simulink library "ADSB_Block"  (R2018b)
settings: Solver=VariableStepAuto  StartTime=0.0  StopTime=10.0  RelTol=1e-3
undefined symbols (not defined in the file): ac1dyn_alt0_ft, ac1dyn_lat0_rad, ac1dyn_lon0_rad, magnitude, uas_adsb_altQuant_ft, uas_adsb_avionicsSeed, uas_adsb_dt_s, uas_adsb_E_bias_ft, uas_adsb_E_random_stddev_ft, uas_adsb_E_tau_s, uas_adsb_Edot_bias_ftps, uas_adsb_Edot_random_stddev_ftps, uas_adsb_Edot_tau_s, uas_adsb_N_bias_ft, uas_adsb_N_random_stddev_ft, uas_adsb_N_tau_s, uas_adsb_Ndot_bias_ftps, uas_adsb_Ndot_random_stddev_ftps, uas_adsb_Ndot_tau_s, uas_adsb_probOneHit_3sec, uas_adsb_probOneHit_7sec, uas_adsb_randProbSeed, uas_adsb_rangeThreshold_ft, uas_adsb_reported_errorCovNED, uas_adsb_seed1, uas_adsb_seed2, uas_adsb_seed3, uas_adsb_seed4, uas_adsb_seed5, uas_adsb_seed6, uas_adsb_seed7, uas_adsb_sns_max_range_ft, uas_adsb_usePerfectAlt
libraries: simulink x7, TSAA_AltRate_Error x1, TSAA_Altitude_Error x1, CreateCovDiagMatrix x1, ExtractCovDiag x1
settings Model: Creator=RA24876  LastModifiedBy=BI28030
settings SFSimCC: SimUseLocalCustomCode=off
settings RTWCC: RTWUseLocalCustomCode=off
settings CodeAppCC: StateflowObjectComments=on

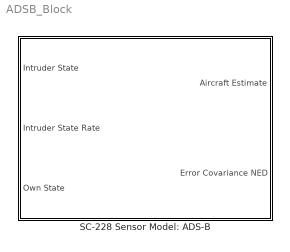
== system ADSB_Block ==
  SC-228 Sensor Model: ADS-B : Subsystem  mask(Tracked Surveillance: ADS-B){var_prefix=int_, dt_s=uas_adsb_dt_s, lat0_rad=ac1dyn_lat0_rad, lon0_rad=ac1dyn_lon0_rad, alt0_ft=ac1dyn_alt0_ft, avionicsSeed=uas_adsb_avionicsSeed, N_random_stddev_ft=uas_adsb_N_random_stddev_ft, N_bias_ft=uas_adsb_N_bias_ft, N_tau_s=uas_adsb_N_tau_s, seed1=uas_adsb_seed1, E_random_stddev_ft=uas_adsb_E_random_stddev_ft, E_bias_ft=uas_adsb_E_bias_ft, E_tau_s=uas_adsb_E_tau_s, seed2=uas_adsb_seed2, Ndot_random_stddev_ftps=uas_adsb_Ndot_random_stddev_ftps, Ndot_bias_ftps=uas_adsb_Ndot_bias_ftps, Ndot_tau_s=uas_adsb_Ndot_tau_s, seed5=uas_adsb_seed5, Edot_random_stddev_ftps=uas_adsb_Edot_random_stddev_ftps, Edot_bias_ftps=uas_adsb_Edot_bias_ftps, Edot_tau_s=uas_adsb_Edot_tau_s, seed6=uas_adsb_seed6, covNED=uas_adsb_reported_errorCovNED, perfect=uas_adsb_usePerfectAlt, seed3=uas_adsb_seed3, seed4=uas_adsb_seed4, altQuant_ft=uas_adsb_altQuant_ft, seed7=uas_adsb_seed7, sns_max_range_ft=uas_adsb_sns_max_range_ft, probOneHit_3sec=uas_adsb_probOneHit_3sec, probOneHit_7sec=uas_adsb_probOneHit_7sec, randProbSeed=uas_adsb_randProbSeed, rangeThreshold_ft=uas_adsb_rangeThreshold_ft}
      mask prompts: var_prefix "Variable Prefix"; dt_s "Timestep"; lat0_rad "ENU Origin Latitude"; lon0_rad "ENU Origin Longitude"; alt0_ft "ENU Origin Altitude"; avionicsSeed "Avionics Delay Seed"; N_random_stddev_ft "North Position Random Error Standard Deviation (ft)"; N_bias_ft "North Position Bias (ft)"; N_tau_s "Correlation Time (s)"; seed1 "Random Seed"; E_random_stddev_ft "East Position Random Error Standard Deviation (ft)"; E_bias_ft "East Position Bias (ft)"; E_tau_s "Correlation Time (s)"; seed2 "Random Seed"; Ndot_random_stddev_ftps "North Velocity Random Error Standard Deviation (ft/s)"; Ndot_bias_ftps "North Velocity Bias (ft/s)"; Ndot_tau_s "Correlation Time (s)"; seed5 "Random Seed"; Edot_random_stddev_ftps "East Velocity Random Error Standard Deviation (ft/s)"; Edot_bias_ftps "East Velocity Bias (ft/s)"; Edot_tau_s "Correlation Time (s)"; seed6 "Random Seed"; covNED "Error Covariance"; perfect "Use Perfect Altimetry"; seed3 "Lambda Random Seed"; seed4 "Random Seed"; altQuant_ft "Altitude Quantization (ft)"; seed7 "Lambda Random Seed"; sns_max_range_ft "Max Detection Range"; probOneHit_3sec "Single Hit Probability (95% detection in 3 sec)"; probOneHit_7sec "Single Hit Probability (95% detection in 7 sec)"; randProbSeed "Random Seed"; rangeThreshold_ft "Range at which detection probabilities change"
      mask help: Additive noise model of ADS-B
      mask init:
      | set_param( [ gcb '/To Workspace' ], 'VariableName', [ var_prefix 'uncompDelay' ] )
      mask Help:
      | Additive noise model of ADS-B. Independent noise is added to each
      | position and velocity component in a North-East-Down coordinate system.
      | Noise is colored using weights determined by time constant parameters.
      | 
      | Output takes the form of a AircraftEstimate data bus and a 6x6 error covariance
      | matrix in North-East-Down.
      mask DialogControl ParameterTabVar0 Prompt: General
      mask DialogControl ParameterTabVar01 Prompt: Position (N)
      mask DialogControl ParameterTabVar012 Prompt: Position (E)
      mask DialogControl ParameterTabVar01234 Prompt: Velocity (N)
      mask DialogControl ParameterTabVar012345 Prompt: Velocity (E)
      mask DialogControl ParameterTabVar01234567 Prompt: Covariance
      mask DialogControl ParameterTabVar012345678 Prompt: Altitude
      mask DialogControl ParameterTabVar0123456789 Prompt: Vertical Rate
      mask DialogControl ParameterTabVar012345678910 Prompt: Detection

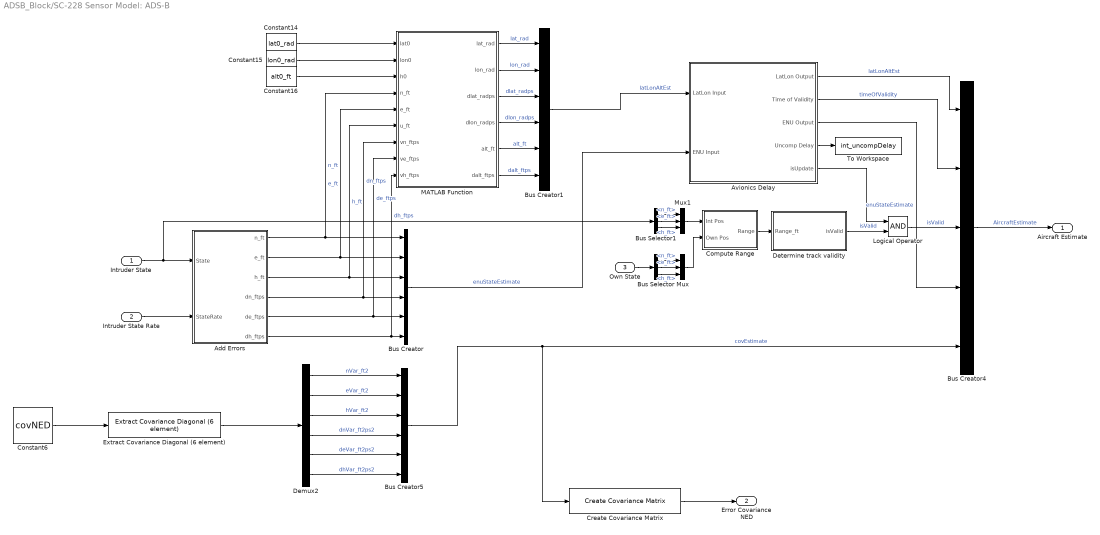
== system ADSB_Block/SC-228 Sensor Model: ADS-B ==
  Intruder State : Inport  OutDataTypeStr=Bus: AircraftState
  Intruder State Rate : Inport  Port=2  OutDataTypeStr=Bus: AircraftStateRate
  Own State : Inport  Port=3  OutDataTypeStr=Bus: AircraftState
  Add Errors : Subsystem
  Avionics Delay : Subsystem  mask{dt=dt_s, seed2=avionicsSeed}
      mask prompts: dt "Sample Time (s)"; seed2 "RNG Seed"
  Bus Creator : BusCreator  Inputs=6  OutDataTypeStr=Bus: StateEstimate
  Bus Creator1 : BusCreator  Inputs=6  OutDataTypeStr=Bus: LatLonAltMeasurement
  Bus Creator4 : BusCreator  Inputs='latLonAltEst','timeOfValidity','isValid','enuStateEstimate','covEstimate'  OutDataTypeStr=Bus: AircraftEstimate  NonVirtualBus=on
  Bus Creator5 : BusCreator  Inputs=6  OutDataTypeStr=Bus: CovarianceEstimate
  Bus Selector : BusSelector  OutputSignals=n_ft,e_ft,h_ft
  Bus Selector1 : BusSelector  OutputSignals=n_ft,e_ft,h_ft
  Compute Range : Subsystem
  Constant14 : Constant  Value=lat0_rad  OutDataTypeStr=double
  Constant15 : Constant  Value=lon0_rad  OutDataTypeStr=double
  Constant16 : Constant  Value=alt0_ft  OutDataTypeStr=double
  Constant6 : Constant  Value=covNED
  Create Covariance Matrix : CreateCovDiagMatrix/Create Covariance Matrix  SystemSampleTime=-1
  Demux2 : Demux  Outputs=6
  Determine track validity : Subsystem  mask{sns_max_range_ft=sns_max_range_ft, probOneHit_3sec=probOneHit_3sec, probOneHit_7sec=probOneHit_7sec, randProbSeed=randProbSeed, rangeThreshold_ft=rangeThreshold_ft}
      mask prompts: sns_max_range_ft "Max Detection Range (ft)"; probOneHit_3sec "Probability of a Single Hit (95% Detection in 3 sec)"; probOneHit_7sec "Probability of a Single Hit (95% Detection in 7 sec)"; randProbSeed "Random Seed"; rangeThreshold_ft "Range Where Detection Probabilites Change"
  Extract Covariance Diagonal (6 element) : ExtractCovDiag/Extract Covariance Diagonal (6 element)  SystemSampleTime=-1
  Logical Operator : Logic  AllPortsSameDT=off  OutDataTypeStr=boolean
  MATLAB Function : MATLAB Function  TreatAsAtomicUnit=on
  Mux : Mux  Inputs=3
  Mux1 : Mux  Inputs=3
  To Workspace : ToWorkspace  VariableName=int_uncompDelay  SaveFormat=Timeseries  SampleTime=-1
  Aircraft Estimate : Outport  OutDataTypeStr=Bus: AircraftEstimate
  Error Covariance NED : Outport  Port=2
  wires:
  Avionics Delay/5(isUpdate) -> Logical Operator/1
  Logical Operator/1 -> Bus Creator4/3  "isValid"
  Mux1/1 -> Compute Range/1(Int Pos)
  Bus Selector1/3 -> Mux1/3  "<h_ft>"
  Bus Selector1/2 -> Mux1/2  "<e_ft>"
  Bus Selector1/1 -> Mux1/1  "<n_ft>"
  Intruder State/1 -> Add Errors/1(State), Bus Selector1/1
  Mux/1 -> Compute Range/2(Own Pos)
  Bus Selector/3 -> Mux/3  "<h_ft>"
  Bus Selector/2 -> Mux/2  "<e_ft>"
  Bus Selector/1 -> Mux/1  "<n_ft>"
  Own State/1 -> Bus Selector/1
  Bus Creator4/1 -> Aircraft Estimate/1  "AircraftEstimate"
  Bus Creator5/1 -> Create Covariance Matrix/1, Bus Creator4/5  "covEstimate"
  MATLAB Function/6(dalt_ftps) -> Bus Creator1/6  "dalt_ftps"
  MATLAB Function/5(alt_ft) -> Bus Creator1/5  "alt_ft"
  MATLAB Function/4(dlon_radps) -> Bus Creator1/4  "dlon_radps"
  MATLAB Function/3(dlat_radps) -> Bus Creator1/3  "dlat_radps"
  MATLAB Function/2(lon_rad) -> Bus Creator1/2  "lon_rad"
  MATLAB Function/1(lat_rad) -> Bus Creator1/1  "lat_rad"
  Bus Creator1/1 -> Avionics Delay/1(LatLon Input)  "latLonAltEst"
  Constant14/1 -> MATLAB Function/1(lat0)
  Constant16/1 -> MATLAB Function/3(h0)
  Constant15/1 -> MATLAB Function/2(lon0)
  Bus Creator/1 -> Avionics Delay/2(ENU Input)  "enuStateEstimate"
  Add Errors/1(n_ft) -> MATLAB Function/4(n_ft), Bus Creator/1  "n_ft"
  Add Errors/2(e_ft) -> MATLAB Function/5(e_ft), Bus Creator/2  "e_ft"
  Add Errors/3(h_ft) -> MATLAB Function/6(u_ft), Bus Creator/3  "h_ft"
  Add Errors/6(dh_ftps) -> MATLAB Function/9(vh_ftps), Bus Creator/6  "dh_ftps"
  Add Errors/4(dn_ftps) -> MATLAB Function/7(vn_ftps), Bus Creator/4  "dn_ftps"
  Add Errors/5(de_ftps) -> MATLAB Function/8(ve_ftps), Bus Creator/5  "de_ftps"
  Intruder State Rate/1 -> Add Errors/2(StateRate)
  Extract Covariance Diagonal (6 element)/1 -> Demux2/1
  Demux2/4 -> Bus Creator5/4  "dnVar_ft2ps2"
  Demux2/5 -> Bus Creator5/5  "deVar_ft2ps2"
  Demux2/2 -> Bus Creator5/2  "eVar_ft2"
  Demux2/1 -> Bus Creator5/1  "nVar_ft2"
  Constant6/1 -> Extract Covariance Diagonal (6 element)/1
  Compute Range/1(Range) -> Determine track validity/1(Range_ft)
  Determine track validity/1(isValid) -> Logical Operator/2  "isValid"
  Avionics Delay/3(ENU Output) -> Bus Creator4/4  "enuStateEstimate"
  Avionics Delay/2(Time of Validity) -> Bus Creator4/2  "timeOfValidity"
  Avionics Delay/4(Uncomp Delay) -> To Workspace/1
  Avionics Delay/1(LatLon Output) -> Bus Creator4/1  "latLonAltEst"
  Demux2/3 -> Bus Creator5/3  "hVar_ft2"
  Demux2/6 -> Bus Creator5/6  "dhVar_ft2ps2"
  Create Covariance Matrix/1 -> Error Covariance NED/1

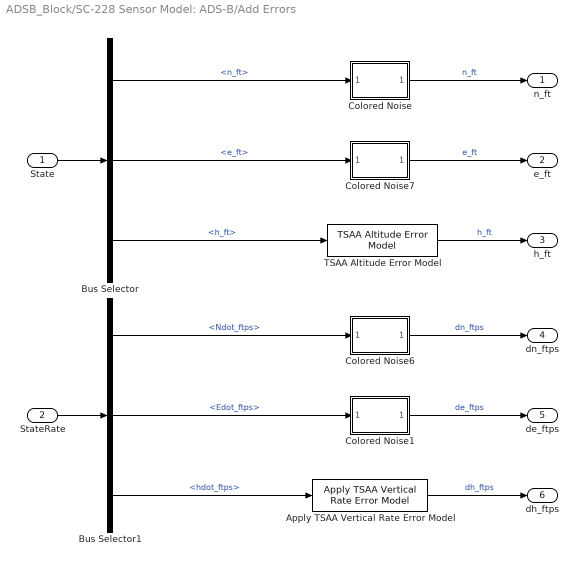
== system ADSB_Block/SC-228 Sensor Model: ADS-B/Add Errors ==
  State : Inport  OutDataTypeStr=Bus: AircraftState
  StateRate : Inport  Port=2  OutDataTypeStr=Bus: AircraftStateRate
  Apply TSAA Vertical Rate Error Model : TSAA_AltRate_Error/Apply TSAA Vertical Rate Error Model  perfect=perfect  seed=seed6  dt_s=dt_s
  Bus Selector : BusSelector  OutputSignals=n_ft,e_ft,h_ft
  Bus Selector1 : BusSelector  OutputSignals=Ndot_ftps,Edot_ftps,hdot_ftps
  Colored Noise : Subsystem  mask(Colored Noise){sig=N_random_stddev_ft, bias=N_bias_ft, tau=N_tau_s, dt=dt_s, seed=seed1}
      mask prompts: sig "Random error standard deviation"; bias "Bias error"; tau "Correlation time"; dt "Track update time"; seed "Random Seed"
      mask help: Generates a noisy state variable estimate using the ABSAA colored noise model. Set correlation time to zero for white noise.
      mask Help:
      | Generates a noisy state variable estimate using the AF Common ABSAA error
      | model.  Time correlation of the error is defined by an exponential decay
      | of K = exp(-tau/dt), where tau is the correlation time and dt is the time
      | between track updates.  The track error at time t is then:
      | 
      |     err(t) = K*err(t-1) + N(0,(1-K^2)*sig^2) + bias
      | 
      | where N(x,y) is a Gaussian noise process with mean x and variance y and
      | with random number generator seeded with the integer 'seed'.
      | 
      | The random noise process must be initialized with an error drawn from
      | N(0,sig^2).
      | 
      | The noise model can be used to produce white noise by setting tau to zero.
  Colored Noise1 : Subsystem  mask(Colored Noise){sig=Edot_random_stddev_ftps, bias=Edot_bias_ftps, tau=Edot_tau_s, dt=dt_s, seed=seed6}
      mask prompts: sig "Random error standard deviation"; bias "Bias error"; tau "Correlation time"; dt "Track update time"; seed "Random Seed"
      mask help: Generates a noisy state variable estimate using the ABSAA colored noise model. Set correlation time to zero for white noise.
      mask Help:
      | Generates a noisy state variable estimate using the AF Common ABSAA error
      | model.  Time correlation of the error is defined by an exponential decay
      | of K = exp(-tau/dt), where tau is the correlation time and dt is the time
      | between track updates.  The track error at time t is then:
      | 
      |     err(t) = K*err(t-1) + N(0,(1-K^2)*sig^2) + bias
      | 
      | where N(x,y) is a Gaussian noise process with mean x and variance y and
      | with random number generator seeded with the integer 'seed'.
      | 
      | The random noise process must be initialized with an error drawn from
      | N(0,sig^2).
      | 
      | The noise model can be used to produce white noise by setting tau to zero.
  Colored Noise6 : Subsystem  mask(Colored Noise){sig=Ndot_random_stddev_ftps, bias=Ndot_bias_ftps, tau=Ndot_tau_s, dt=dt_s, seed=seed5}
      mask prompts: sig "Random error standard deviation"; bias "Bias error"; tau "Correlation time"; dt "Track update time"; seed "Random Seed"
      mask help: Generates a noisy state variable estimate using the ABSAA colored noise model. Set correlation time to zero for white noise.
      mask Help:
      | Generates a noisy state variable estimate using the AF Common ABSAA error
      | model.  Time correlation of the error is defined by an exponential decay
      | of K = exp(-tau/dt), where tau is the correlation time and dt is the time
      | between track updates.  The track error at time t is then:
      | 
      |     err(t) = K*err(t-1) + N(0,(1-K^2)*sig^2) + bias
      | 
      | where N(x,y) is a Gaussian noise process with mean x and variance y and
      | with random number generator seeded with the integer 'seed'.
      | 
      | The random noise process must be initialized with an error drawn from
      | N(0,sig^2).
      | 
      | The noise model can be used to produce white noise by setting tau to zero.
  Colored Noise7 : Subsystem  mask(Colored Noise){sig=E_random_stddev_ft, bias=E_bias_ft, tau=E_tau_s, dt=dt_s, seed=seed2}
      mask prompts: sig "Random error standard deviation"; bias "Bias error"; tau "Correlation time"; dt "Track update time"; seed "Random Seed"
      mask help: Generates a noisy state variable estimate using the ABSAA colored noise model. Set correlation time to zero for white noise.
      mask Help:
      | Generates a noisy state variable estimate using the AF Common ABSAA error
      | model.  Time correlation of the error is defined by an exponential decay
      | of K = exp(-tau/dt), where tau is the correlation time and dt is the time
      | between track updates.  The track error at time t is then:
      | 
      |     err(t) = K*err(t-1) + N(0,(1-K^2)*sig^2) + bias
      | 
      | where N(x,y) is a Gaussian noise process with mean x and variance y and
      | with random number generator seeded with the integer 'seed'.
      | 
      | The random noise process must be initialized with an error drawn from
      | N(0,sig^2).
      | 
      | The noise model can be used to produce white noise by setting tau to zero.
  TSAA Altitude Error Model : TSAA_Altitude_Error/TSAA Altitude Error Model  ac_id=2  perfect=perfect  lambdaSeed=seed3  randomSeed=seed4  altQuant_ft=altQuant_ft  dt_s=dt_s
  n_ft : Outport
  e_ft : Outport  Port=2
  h_ft : Outport  Port=3
  dn_ftps : Outport  Port=4
  de_ftps : Outport  Port=5
  dh_ftps : Outport  Port=6
  wires:
  Bus Selector/3 -> TSAA Altitude Error Model/1  "<h_ft>"
  Bus Selector/1 -> Colored Noise/1(truth)  "<n_ft>"
  State/1 -> Bus Selector/1
  Colored Noise1/1(noisy) -> de_ftps/1  "de_ftps"
  Apply TSAA Vertical Rate Error Model/1 -> dh_ftps/1  "dh_ftps"
  Colored Noise6/1(noisy) -> dn_ftps/1  "dn_ftps"
  Colored Noise7/1(noisy) -> e_ft/1  "e_ft"
  Colored Noise/1(noisy) -> n_ft/1  "n_ft"
  Bus Selector/2 -> Colored Noise7/1(truth)  "<e_ft>"
  TSAA Altitude Error Model/1 -> h_ft/1  "h_ft"
  StateRate/1 -> Bus Selector1/1
  Bus Selector1/1 -> Colored Noise6/1(truth)  "<Ndot_ftps>"
  Bus Selector1/2 -> Colored Noise1/1(truth)  "<Edot_ftps>"
  Bus Selector1/3 -> Apply TSAA Vertical Rate Error Model/1  "<hdot_ftps>"

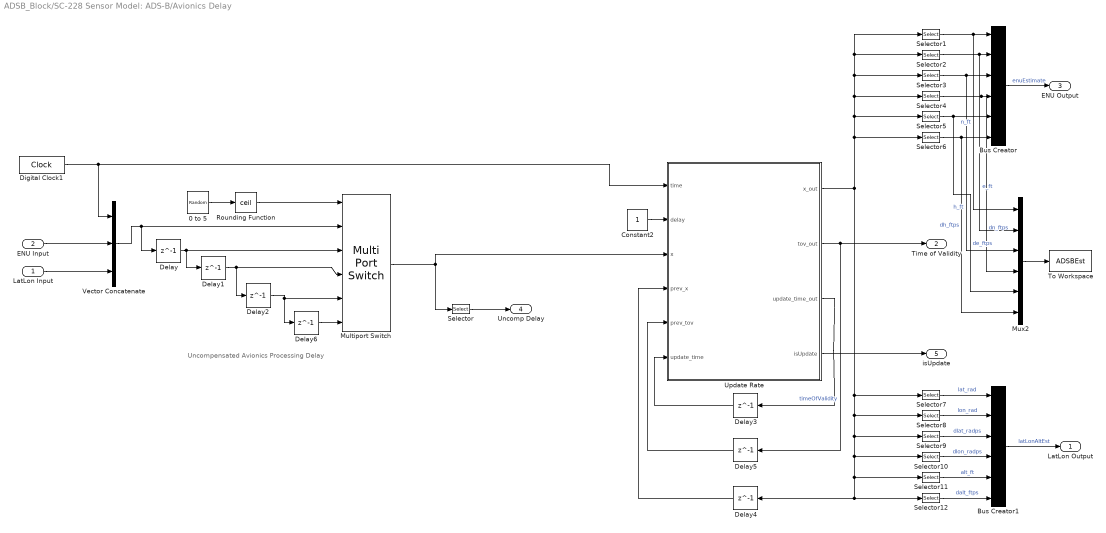
== system ADSB_Block/SC-228 Sensor Model: ADS-B/Avionics Delay ==
  note: Uncompensated Avionics Processing Delay
  LatLon Input : Inport
  ENU Input : Inport  Port=2
  0 to 5 : UniformRandomNumber  Minimum=0  Maximum=5  Seed=seed2  SampleTime=dt_s
  Bus Creator : BusCreator  Inputs=6
  Bus Creator1 : BusCreator  Inputs=6
  Constant2 : Constant
  Delay{,1..2,6} (4 alike) : Delay  DelayLength=1
  Delay3 : Delay  DelayLength=1  InitialCondition=1
  Delay4 : Delay  DelayLength=1  InitialCondition=0
  Delay5 : Delay  DelayLength=1  InitialCondition=0
  Digital Clock1 : DigitalClock  SampleTime=dt_s
  Multiport Switch : MultiPortSwitch  Inputs=5
  Mux2 : Mux  Inputs=6
  Rounding Function : Rounding  Operator=ceil
  Selector : Selector  InputPortWidth=13  IndexOptions=Index vector (dialog)  Indices=[1]  OutputSizes=1
  Selector1 : Selector  InputPortWidth=13  IndexOptions=Index vector (dialog)  Indices=[2]  OutputSizes=1
  Selector10 : Selector  InputPortWidth=13  IndexOptions=Index vector (dialog)  Indices=[11]  OutputSizes=1
  Selector11 : Selector  InputPortWidth=13  IndexOptions=Index vector (dialog)  Indices=[12]  OutputSizes=1
  Selector12 : Selector  InputPortWidth=13  IndexOptions=Index vector (dialog)  Indices=[13]  OutputSizes=1
  Selector2 : Selector  InputPortWidth=13  IndexOptions=Index vector (dialog)  Indices=[3]  OutputSizes=1
  Selector3 : Selector  InputPortWidth=13  IndexOptions=Index vector (dialog)  Indices=[4]  OutputSizes=1
  Selector4 : Selector  InputPortWidth=13  IndexOptions=Index vector (dialog)  Indices=[5]  OutputSizes=1
  Selector5 : Selector  InputPortWidth=13  IndexOptions=Index vector (dialog)  Indices=[6]  OutputSizes=1
  Selector6 : Selector  InputPortWidth=13  IndexOptions=Index vector (dialog)  Indices=[7]  OutputSizes=1
  Selector7 : Selector  InputPortWidth=13  IndexOptions=Index vector (dialog)  Indices=[8]  OutputSizes=1
  Selector8 : Selector  InputPortWidth=13  IndexOptions=Index vector (dialog)  Indices=[9]  OutputSizes=1
  Selector9 : Selector  InputPortWidth=13  IndexOptions=Index vector (dialog)  Indices=[10]  OutputSizes=1
  To Workspace : ToWorkspace  VariableName=ADSBEst  SampleTime=-1
  Update Rate : MATLAB Function  TreatAsAtomicUnit=on
  Vector Concatenate : Concatenate  NumInputs=3
  LatLon Output : Outport
  Time of Validity : Outport  Port=2
  ENU Output : Outport  Port=3
  Uncomp Delay : Outport  Port=4
  isUpdate : Outport  Port=5
  wires:
  Update Rate/4(isUpdate) -> isUpdate/1
  Constant2/1 -> Update Rate/2(delay)
  Selector1/1 -> Mux2/1, Bus Creator/1  "n_ft"
  Vector Concatenate/1 -> Delay/1, Multiport Switch/2
  Selector/1 -> Uncomp Delay/1
  ENU Input/1 -> Vector Concatenate/2
  Multiport Switch/1 -> Update Rate/3(x), Selector/1
  Delay5/1 -> Update Rate/5(prev_tov)
  Update Rate/2(tov_out) -> Time of Validity/1, Delay5/1  "timeOfValidity"
  Delay3/1 -> Update Rate/6(update_time)
  Delay4/1 -> Update Rate/4(prev_x)
  Update Rate/3(update_time_out) -> Delay3/1
  Digital Clock1/1 -> Update Rate/1(time), Vector Concatenate/1
  Rounding Function/1 -> Multiport Switch/1
  0 to 5/1 -> Rounding Function/1
  Delay/1 -> Multiport Switch/3, Delay1/1
  Delay1/1 -> Multiport Switch/4, Delay2/1
  Delay2/1 -> Multiport Switch/5, Delay6/1
  Selector2/1 -> Mux2/2, Bus Creator/2  "e_ft"
  Selector3/1 -> Mux2/3, Bus Creator/3  "h_ft"
  Selector4/1 -> Mux2/4, Bus Creator/4  "dn_ftps"
  Selector5/1 -> Mux2/5, Bus Creator/5  "de_ftps"
  Selector6/1 -> Mux2/6, Bus Creator/6  "dh_ftps"
  Bus Creator/1 -> ENU Output/1  "enuEstimate"
  Delay6/1 -> Multiport Switch/6
  LatLon Input/1 -> Vector Concatenate/3
  Bus Creator1/1 -> LatLon Output/1  "latLonAltEst"
  Update Rate/1(x_out) -> Selector7/1, Delay4/1, Selector12/1, Selector11/1, Selector10/1, Selector9/1, Selector8/1, Selector6/1, Selector5/1, Selector4/1, Selector3/1, Selector2/1, Selector1/1
  Selector12/1 -> Bus Creator1/6  "dalt_ftps"
  Selector7/1 -> Bus Creator1/1  "lat_rad"
  Selector8/1 -> Bus Creator1/2  "lon_rad"
  Selector11/1 -> Bus Creator1/5  "alt_ft"
  Selector10/1 -> Bus Creator1/4  "dlon_radps"
  Selector9/1 -> Bus Creator1/3  "dlat_radps"
  Mux2/1 -> To Workspace/1

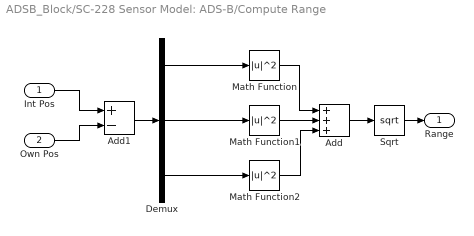
== system ADSB_Block/SC-228 Sensor Model: ADS-B/Compute Range ==
  Int Pos : Inport
  Own Pos : Inport  Port=2
  Add : Sum  Inputs=+++
  Add1 : Sum  Inputs=+-
  Demux : Demux  Outputs=3
  Math Function : Math  Operator=magnitude^2  SaturateOnIntegerOverflow=on
  Math Function1 : Math  Operator=magnitude^2  SaturateOnIntegerOverflow=on
  Math Function2 : Math  Operator=magnitude^2  SaturateOnIntegerOverflow=on
  Sqrt : Sqrt  SaturateOnIntegerOverflow=on
  Range : Outport
  wires:
  Demux/3 -> Math Function2/1
  Demux/1 -> Math Function/1
  Demux/2 -> Math Function1/1
  Add1/1 -> Demux/1
  Own Pos/1 -> Add1/2
  Int Pos/1 -> Add1/1
  Math Function/1 -> Add/1
  Sqrt/1 -> Range/1
  Math Function1/1 -> Add/2
  Add/1 -> Sqrt/1
  Math Function2/1 -> Add/3

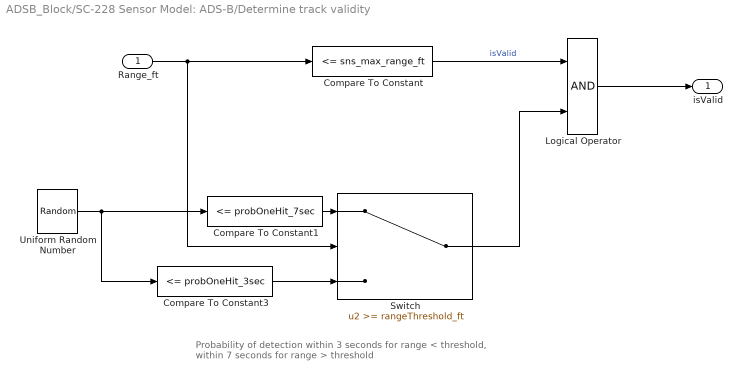
== system ADSB_Block/SC-228 Sensor Model: ADS-B/Determine track validity ==
  note: Probability of detection within 3 seconds for range < threshold,
      | within 7 seconds for range > threshold
  Range_ft : Inport
  Compare To Constant : simulink/Logic and Bit Operations/Compare To Constant  relop=<=  const=sns_max_range_ft  OutDataTypeStr=boolean
  Compare To Constant1 : simulink/Logic and Bit Operations/Compare To Constant  relop=<=  const=probOneHit_7sec  OutDataTypeStr=boolean
  Compare To Constant3 : simulink/Logic and Bit Operations/Compare To Constant  relop=<=  const=probOneHit_3sec  OutDataTypeStr=boolean
  Logical Operator : Logic  AllPortsSameDT=off  OutDataTypeStr=boolean
  Switch : Switch  Threshold=rangeThreshold_ft
  Uniform Random Number : UniformRandomNumber  Minimum=0  Seed=randProbSeed  SampleTime=dt_s
  isValid : Outport
  wires:
  Range_ft/1 -> Compare To Constant/1, Switch/2
  Compare To Constant/1 -> Logical Operator/1  "isValid"
  Logical Operator/1 -> isValid/1
  Switch/1 -> Logical Operator/2
  Compare To Constant1/1 -> Switch/1
  Uniform Random Number/1 -> Compare To Constant3/1, Compare To Constant1/1
  Compare To Constant3/1 -> Switch/3

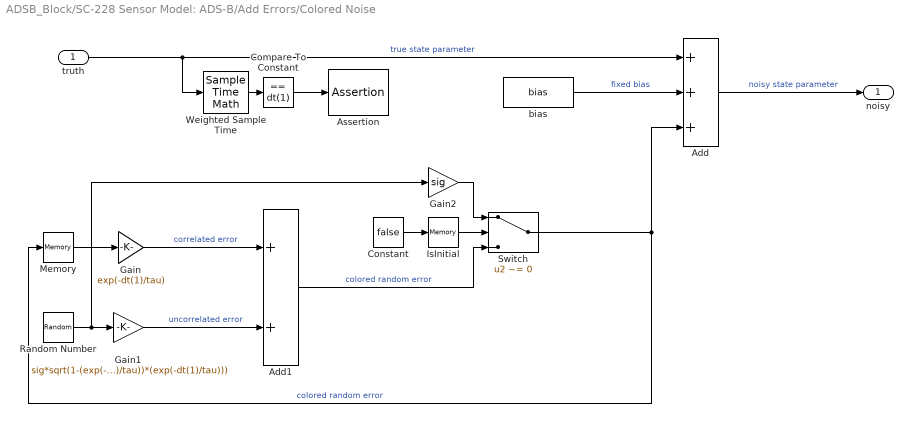
== system ADSB_Block/SC-228 Sensor Model: ADS-B/Add Errors/Colored Noise ==
  truth : Inport
  Add : Sum  Inputs=+++
  Add1 : Sum
  Assertion : Assertion
  Compare To Constant : simulink/Logic and Bit Operations/Compare To Constant  relop===  const=dt(1)  OutDataTypeStr=boolean
  Constant : Constant  Value=false
  Gain : Gain  Gain=exp(-dt(1)/tau)
  Gain1 : Gain  Gain=sig*sqrt(1-(exp(-dt(1)/tau))*(exp(-dt(1)/tau)))
  Gain2 : Gain  Gain=sig
  IsInitial : Memory  InitialCondition=true  InheritSampleTime=on
  Memory : Memory  InheritSampleTime=on
  Random Number : RandomNumber  Seed=seed  SampleTime=dt_s
  Switch : Switch  Criteria=u2 ~= 0
  Weighted Sample Time : SampleTimeMath  TsampMathOp=Ts Only
  bias : Constant  Value=bias
  noisy : Outport
  wires:
  Compare To Constant/1 -> Assertion/1
  Weighted Sample Time/1 -> Compare To Constant/1
  Gain2/1 -> Switch/1
  Add1/1 -> Switch/3  "colored random error"
  IsInitial/1 -> Switch/2
  Constant/1 -> IsInitial/1
  Memory/1 -> Gain/1
  truth/1 -> Add/1, Weighted Sample Time/1  "true state parameter"
  Add/1 -> noisy/1  "noisy state parameter"
  Gain/1 -> Add1/1  "correlated error"
  Random Number/1 -> Gain1/1, Gain2/1
  bias/1 -> Add/2  "fixed bias"
  Switch/1 -> Add/3, Memory/1  "colored random error"
  Gain1/1 -> Add1/2  "uncorrelated error"

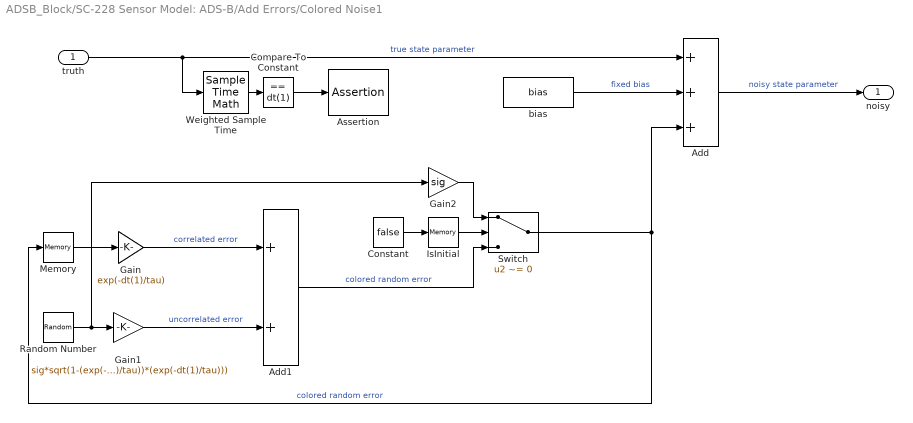
== system ADSB_Block/SC-228 Sensor Model: ADS-B/Add Errors/Colored Noise1 ==
  truth : Inport
  Add : Sum  Inputs=+++
  Add1 : Sum
  Assertion : Assertion
  Compare To Constant : simulink/Logic and Bit Operations/Compare To Constant  relop===  const=dt(1)  OutDataTypeStr=boolean
  Constant : Constant  Value=false
  Gain : Gain  Gain=exp(-dt(1)/tau)
  Gain1 : Gain  Gain=sig*sqrt(1-(exp(-dt(1)/tau))*(exp(-dt(1)/tau)))
  Gain2 : Gain  Gain=sig
  IsInitial : Memory  InitialCondition=true  InheritSampleTime=on
  Memory : Memory  InheritSampleTime=on
  Random Number : RandomNumber  Seed=seed  SampleTime=dt_s
  Switch : Switch  Criteria=u2 ~= 0
  Weighted Sample Time : SampleTimeMath  TsampMathOp=Ts Only
  bias : Constant  Value=bias
  noisy : Outport
  wires:
  Compare To Constant/1 -> Assertion/1
  Weighted Sample Time/1 -> Compare To Constant/1
  Gain2/1 -> Switch/1
  Add1/1 -> Switch/3  "colored random error"
  IsInitial/1 -> Switch/2
  Constant/1 -> IsInitial/1
  Memory/1 -> Gain/1
  truth/1 -> Add/1, Weighted Sample Time/1  "true state parameter"
  Add/1 -> noisy/1  "noisy state parameter"
  Gain/1 -> Add1/1  "correlated error"
  Random Number/1 -> Gain1/1, Gain2/1
  bias/1 -> Add/2  "fixed bias"
  Switch/1 -> Add/3, Memory/1  "colored random error"
  Gain1/1 -> Add1/2  "uncorrelated error"

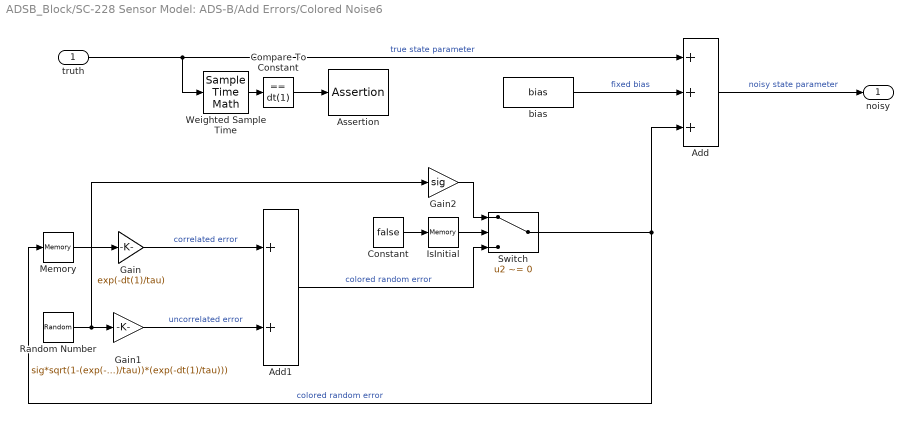
== system ADSB_Block/SC-228 Sensor Model: ADS-B/Add Errors/Colored Noise6 ==
  truth : Inport
  Add : Sum  Inputs=+++
  Add1 : Sum
  Assertion : Assertion
  Compare To Constant : simulink/Logic and Bit Operations/Compare To Constant  relop===  const=dt(1)  OutDataTypeStr=boolean
  Constant : Constant  Value=false
  Gain : Gain  Gain=exp(-dt(1)/tau)
  Gain1 : Gain  Gain=sig*sqrt(1-(exp(-dt(1)/tau))*(exp(-dt(1)/tau)))
  Gain2 : Gain  Gain=sig
  IsInitial : Memory  InitialCondition=true  InheritSampleTime=on
  Memory : Memory  InheritSampleTime=on
  Random Number : RandomNumber  Seed=seed  SampleTime=dt_s
  Switch : Switch  Criteria=u2 ~= 0
  Weighted Sample Time : SampleTimeMath  TsampMathOp=Ts Only
  bias : Constant  Value=bias
  noisy : Outport
  wires:
  Compare To Constant/1 -> Assertion/1
  Weighted Sample Time/1 -> Compare To Constant/1
  Gain2/1 -> Switch/1
  Add1/1 -> Switch/3  "colored random error"
  IsInitial/1 -> Switch/2
  Constant/1 -> IsInitial/1
  Memory/1 -> Gain/1
  truth/1 -> Add/1, Weighted Sample Time/1  "true state parameter"
  Add/1 -> noisy/1  "noisy state parameter"
  Gain/1 -> Add1/1  "correlated error"
  Random Number/1 -> Gain1/1, Gain2/1
  bias/1 -> Add/2  "fixed bias"
  Switch/1 -> Add/3, Memory/1  "colored random error"
  Gain1/1 -> Add1/2  "uncorrelated error"

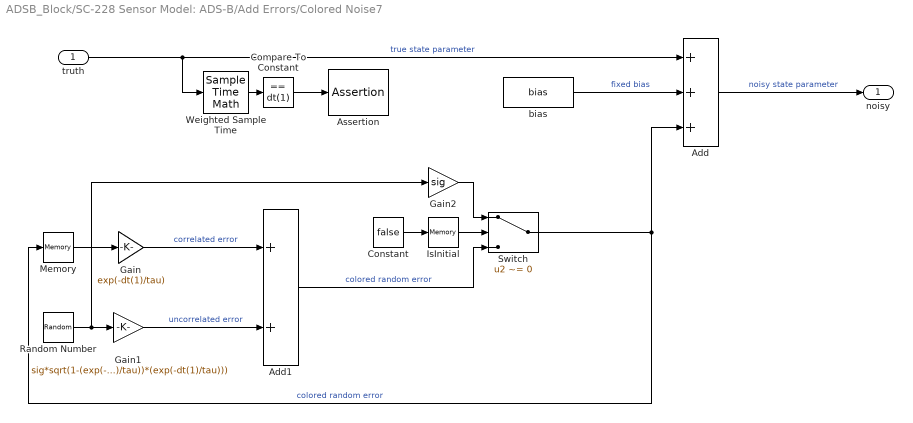
== system ADSB_Block/SC-228 Sensor Model: ADS-B/Add Errors/Colored Noise7 ==
  truth : Inport
  Add : Sum  Inputs=+++
  Add1 : Sum
  Assertion : Assertion
  Compare To Constant : simulink/Logic and Bit Operations/Compare To Constant  relop===  const=dt(1)  OutDataTypeStr=boolean
  Constant : Constant  Value=false
  Gain : Gain  Gain=exp(-dt(1)/tau)
  Gain1 : Gain  Gain=sig*sqrt(1-(exp(-dt(1)/tau))*(exp(-dt(1)/tau)))
  Gain2 : Gain  Gain=sig
  IsInitial : Memory  InitialCondition=true  InheritSampleTime=on
  Memory : Memory  InheritSampleTime=on
  Random Number : RandomNumber  Seed=seed  SampleTime=dt_s
  Switch : Switch  Criteria=u2 ~= 0
  Weighted Sample Time : SampleTimeMath  TsampMathOp=Ts Only
  bias : Constant  Value=bias
  noisy : Outport
  wires:
  Gain1/1 -> Add1/2  "uncorrelated error"
  Switch/1 -> Memory/1, Add/3  "colored random error"
  bias/1 -> Add/2  "fixed bias"
  Random Number/1 -> Gain2/1, Gain1/1
  Gain/1 -> Add1/1  "correlated error"
  Add/1 -> noisy/1  "noisy state parameter"
  truth/1 -> Weighted Sample Time/1, Add/1  "true state parameter"
  Memory/1 -> Gain/1
  Constant/1 -> IsInitial/1
  IsInitial/1 -> Switch/2
  Add1/1 -> Switch/3  "colored random error"
  Gain2/1 -> Switch/1
  Weighted Sample Time/1 -> Compare To Constant/1
  Compare To Constant/1 -> Assertion/1

== matlab function ADSB_Block/SC-228 Sensor Model: ADS-B/Avionics Delay/Update Rate ==
  data: time input; x_out output; tov_out output; delay input; x input; prev_x input; prev_tov input; update_time input; update_time_out output; isUpdate output
function [x_out,tov_out,update_time_out,isUpdate] = fcn(time,delay,x,prev_x,prev_tov,update_time)
%#codegen

if time-update_time>=-0.001 % pass out new output
    update_time_out = time+delay; 
    x_out = x;
    tov_out = time;
    isUpdate = true;
else % continue passing out old output
    x_out = prev_x; 
    update_time_out = update_time;
    tov_out = prev_tov;
    isUpdate = false;
end

== matlab function ADSB_Block/SC-228 Sensor Model: ADS-B/MATLAB Function ==
  data: lat0 input double; lon0 input double; h0 input double; n_ft input double; e_ft input double size=1; u_ft input double; vn_ftps input double; ve_ftps input double; vh_ftps input double; lat_rad output double; lon_rad output double; dlat_radps output double; dlon_radps output double; alt_ft output double; dalt_ftps output double
function [lat_rad,lon_rad,dlat_radps,dlon_radps,alt_ft,dalt_ftps] = convertToLLA(lat0,lon0,h0,n_ft,e_ft,u_ft,vn_ftps,ve_ftps,vh_ftps)
%#codegen

% WGS-84 ellipsoid constants
a = 2.09256*10^7;          %Semi-major axis (meters)
f = 1.0/298.257223563;  %Flattening
ecc_sq = f*(2.0-f);        %Eccentricity^2


% Ellipsoidal "radius"
er = a./sqrt(1-ecc_sq.*sin(lat0).^2);


% ECEF coordinates
x0 = (er + h0)*cos(lat0)*cos(lon0);
y0 = (er + h0)*cos(lat0)*sin(lon0);
z0 = (er.*(1-ecc_sq) + h0)*sin(lat0);


%% Rotation Matrix
posECEF0 = [x0;y0;z0];
% Compute the local Up unit vector
vHatU = posECEF0;
vHatU(3) = vHatU(3) ./ ((1-f)^2);
vHatU = vHatU ./ norm(vHatU);

% Compute the projection onto the local Up vector
pU = vHatU * vHatU';

% Compute the projection onto the local Tangent plane
pT = eye(size(pU)) - pU;

% Compute the local North unit vector
vHatZ = [0;0;1];
vHatN = pT * vHatZ;
vHatN = vHatN ./ norm(vHatN);

% Compute the local East unit vector
vHatE = cross(vHatN,vHatU);

% Compute ENU rotation matrix
rotMatENU = zeros(3,3);
rotMatENU(:,1) = vHatE;
rotMatENU(:,2) = vHatN;
rotMatENU(:,3) = vHatU;

tPosECEF = rotMatENU*[e_ft;n_ft;u_ft] + [x0;y0;z0];


%% ECEF to LLA
% WGS-84 derived parameters
b = (1-f).*a;                       %Semi-minor axis (meters)
ecc1_sq = (a.^2 - b.^2)./(a.^2);    %First eccentricity squared
ecc2_sq = (a.^2 - b.^2)./(b.^2);    %Second eccentricity squared


% Length of position vector in equatorial plane
rho = sqrt(tPosECEF(1).^2 + tPosECEF(2).^2);

% Auxillary angle
theta = atan( (tPosECEF(3).*a)./(rho.*b) );

lon_rad = atan2(tPosECEF(2),tPosECEF(1));
lat_rad = atan( (tPosECEF(3) + ecc2_sq.*b.*(sin(theta)).^3)./(rho - ecc1_sq.*a.*(cos(theta)).^3) );

ewRadCurv = a./sqrt(1-ecc1_sq.*sin(lat_rad).^2);

alt_ft = (rho./cos(lat_rad)) - ewRadCurv;


%% Velocities - Project 1 sec into future and use to estimate
dalt_ftps = vh_ftps; % Assume about the same


tPosECEF_1sec = rotMatENU*[e_ft+ve_ftps;...
                           n_ft+vn_ftps;...
                           u_ft] + ...
                           [x0;y0;z0];

% Length of position vector in equatorial plane
rho = sqrt(tPosECEF_1sec(1).^2 + tPosECEF_1sec(2).^2);

% Auxillary angle
theta = atan( (tPosECEF_1sec(3).*a)./(rho.*b) );

lon_rad_1sec = atan2(tPosECEF_1sec(2),tPosECEF_1sec(1));
lat_rad_1sec = atan( (tPosECEF_1sec(3) + ecc2_sq.*b.*(sin(theta)).^3)./(rho - ecc1_sq.*a.*(cos(theta)).^3) );

dlat_radps = lat_rad_1sec - lat_rad;
dlon_radps = lon_rad_1sec - lon_rad;
end
